simulink model "trial"  (R2020b)
settings: Solver=VariableStepAuto  StartTime=0.0  StopTime=10.0  RelTol=1e-3
libraries: simulink x2
settings Model: Creator=99003785  LastModifiedBy=99003785

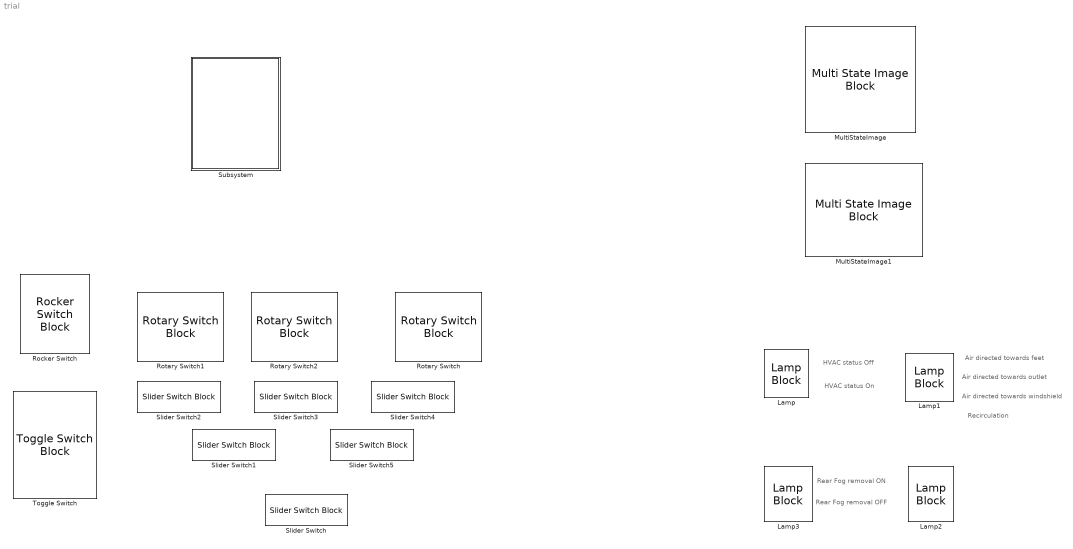
== system trial ==
  note: Rear Fog removal OFF
  note: Recirculation
  note: Air directed towards feet
  note: Air directed towards outlet
  note: Air directed towards windshield
  note: HVAC status On
  note: Rear Fog removal ON
  note: HVAC status Off
  Lamp{,1..3} (4 alike) : LampBlock
  MultiStateImage : MultiStateImageBlock
  MultiStateImage1 : MultiStateImageBlock
  Rocker Switch : RockerSwitchBlock
      settings: Values={{'On', 'Off'}, [1 0]}
  Rotary Switch : RotarySwitchBlock
      settings: Values={{'Off', 'Low', 'Medium', 'High'}, [0 1 2 3]}
  Rotary Switch1 : RotarySwitchBlock
      settings: Values={{'Off', 'Low', 'Medium', 'High'}, [0 1 2 3]}
  Rotary Switch2 : RotarySwitchBlock
      settings: Values={{'Off', 'AC', 'Heater', 'Air-Vent'}, [0 1 2 3]}
  Slider Switch{,1..5} (6 alike) : SliderSwitchBlock
      settings: Values={{'Off', 'On'}, [0 1]}
  Subsystem : Subsystem
  Toggle Switch : ToggleSwitchBlock
      settings: Values={{'Off', 'On'}, [0 1]}

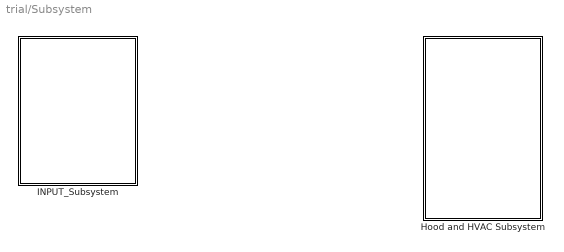
== system trial/Subsystem ==
  Hood and HVAC Subsystem : Subsystem  TreatAsAtomicUnit=on
  INPUT_Subsystem : Subsystem

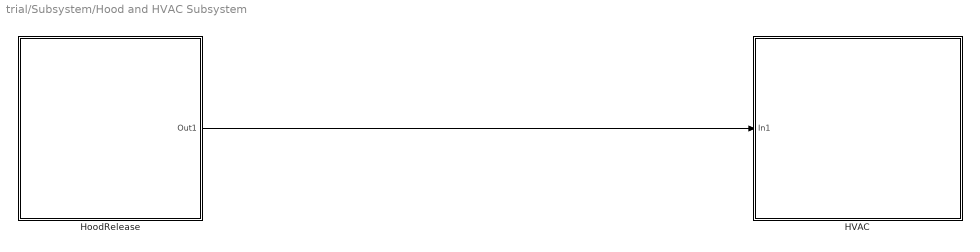
== system trial/Subsystem/Hood and HVAC Subsystem ==
  HVAC : Subsystem
  HoodRelease : Subsystem
  wires:
  HoodRelease/1(Out1) -> HVAC/1(In1)

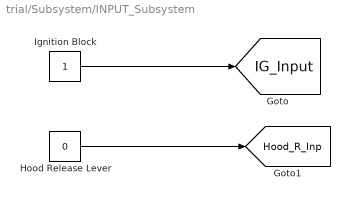
== system trial/Subsystem/INPUT_Subsystem ==
  Hood Release Lever : Constant  Value=0
  Ignition Block : Constant
  tag scope: Hood_R_Inp=global, IG_Input=global
  wires:
  Ignition Block/1 -> [IG_Input]
  Hood Release Lever/1 -> [Hood_R_Inp]

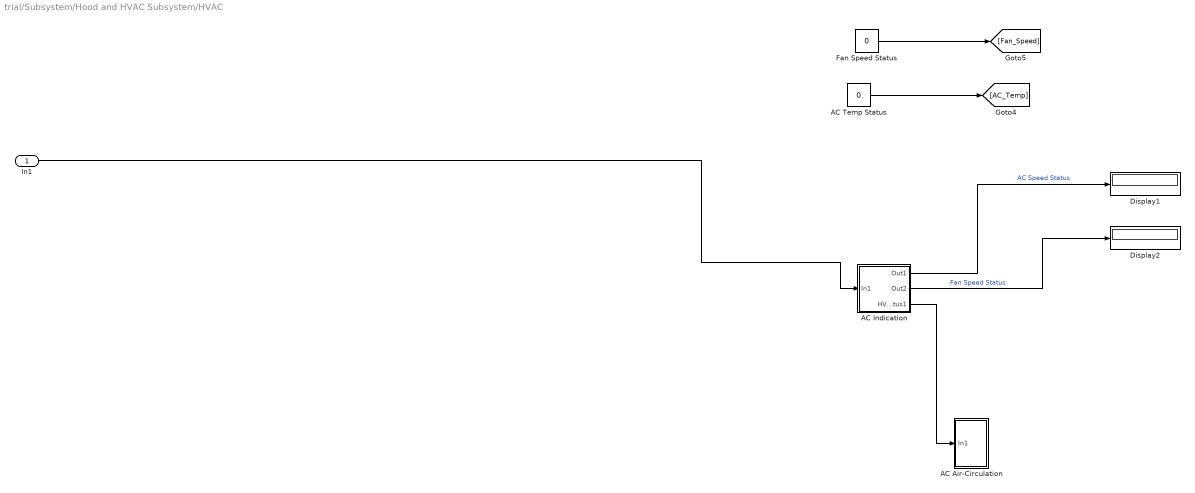
== system trial/Subsystem/Hood and HVAC Subsystem/HVAC ==
  In1 : Inport
  AC Air-Circulation : Subsystem
  AC Indication : Subsystem
  AC Temp Status : Constant  Value=0
  Display1 : Display
  Display2 : Display
  Fan Speed Status : Constant  Value=0
  wires:
  In1/1 -> AC Indication/1(In1)
  AC Indication/1(Out1) -> Display1/1  "AC Speed Status"
  AC Indication/2(Out2) -> Display2/1  "Fan Speed Status"
  AC Indication/3(HVAC Status1) -> AC Air-Circulation/1(In1)
  Fan Speed Status/1 -> [Fan_Speed]
  AC Temp Status/1 -> [AC_Temp]

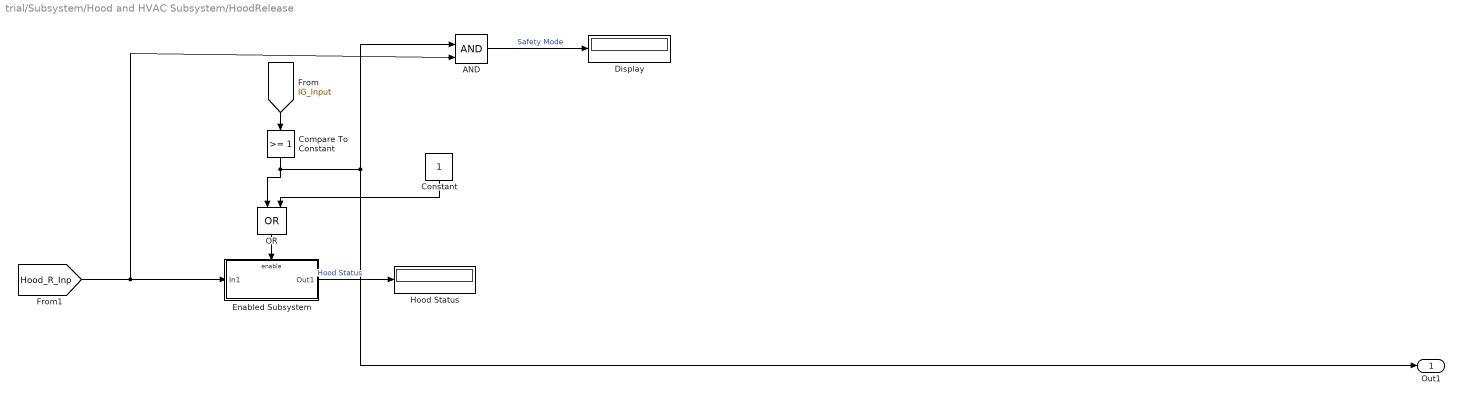
== system trial/Subsystem/Hood and HVAC Subsystem/HoodRelease ==
  AND : Logic  IconShape=distinctive  AllPortsSameDT=off  OutDataTypeStr=boolean
  Compare To Constant : simulink/Logic and Bit Operations/Compare To Constant  relop=>=  const=1  OutDataTypeStr=boolean
  Constant : Constant
  Display : Display
  Enabled Subsystem : Subsystem  TreatAsAtomicUnit=on
  Hood Status : Display
  OR : Logic  Operator=OR  IconShape=distinctive  AllPortsSameDT=off  OutDataTypeStr=boolean
  Out1 : Outport
  wires:
  [Hood_R_Inp] -> AND/2, Enabled Subsystem/1(In1)
  Enabled Subsystem/1(Out1) -> Hood Status/1  "Hood Status"
  Constant/1 -> OR/2
  OR/1 -> Enabled Subsystem/Enable
  AND/1 -> Display/1  "Safety Mode"
  [IG_Input] -> Compare To Constant/1
  Compare To Constant/1 -> Out1/1, AND/1, OR/1

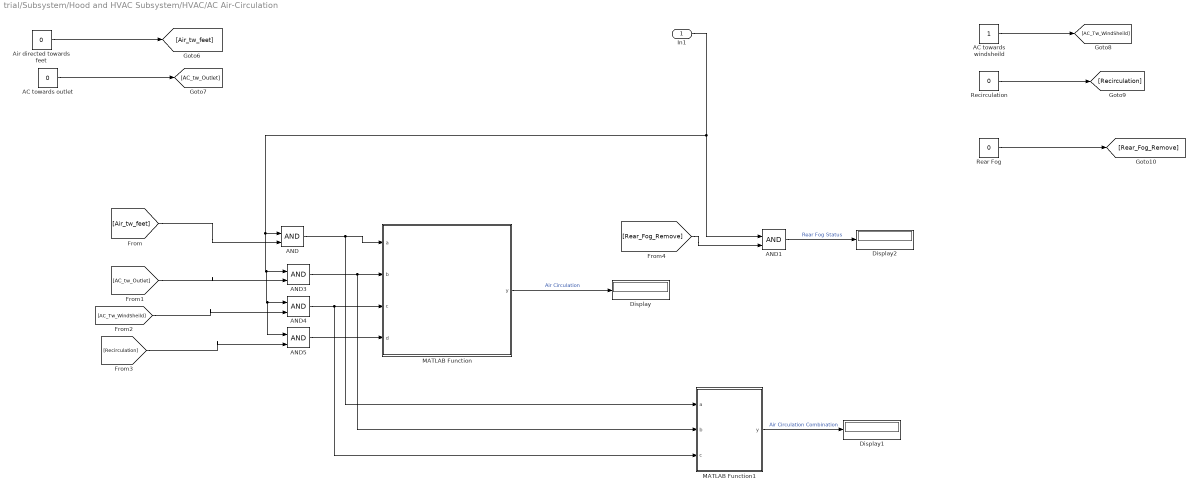
== system trial/Subsystem/Hood and HVAC Subsystem/HVAC/AC Air-Circulation ==
  In1 : Inport
  AC towards outlet : Constant  Value=0
  AC towards windsheild : Constant
  AND{,1,3..5} (5 alike) : Logic  IconShape=distinctive  AllPortsSameDT=off  OutDataTypeStr=boolean
  Air directed towards feet : Constant  Value=0
  Display : Display
  Display1 : Display
  Display2 : Display
  MATLAB Function : MATLAB Function  TreatAsAtomicUnit=on
  MATLAB Function1 : MATLAB Function  TreatAsAtomicUnit=on
  Rear Fog : Constant  Value=0
  Recirculation : Constant  Value=0
  wires:
  [AC_tw_Outlet] -> AND3/2
  In1/1 -> AND1/1, AND5/1, AND4/1, AND3/1, AND/1
  AND4/1 -> MATLAB Function1/3(c), MATLAB Function/3(c)
  MATLAB Function/1(y) -> Display/1  "Air Circulation"
  AND/1 -> MATLAB Function1/1(a), MATLAB Function/1(a)
  AND3/1 -> MATLAB Function1/2(b), MATLAB Function/2(b)
  AND5/1 -> MATLAB Function/4(d)
  [Air_tw_feet] -> AND/2
  MATLAB Function1/1(y) -> Display1/1  "Air Circulation Combination"
  [Rear_Fog_Remove] -> AND1/2
  AND1/1 -> Display2/1  "Rear Fog Status"
  [AC_Tw_WindSheild] -> AND4/2
  [Recirculation] -> AND5/2
  Air directed towards feet/1 -> [Air_tw_feet]
  AC towards outlet/1 -> [AC_tw_Outlet]
  Rear Fog/1 -> [Rear_Fog_Remove]
  Recirculation/1 -> [Recirculation]
  AC towards windsheild/1 -> [AC_Tw_WindSheild]

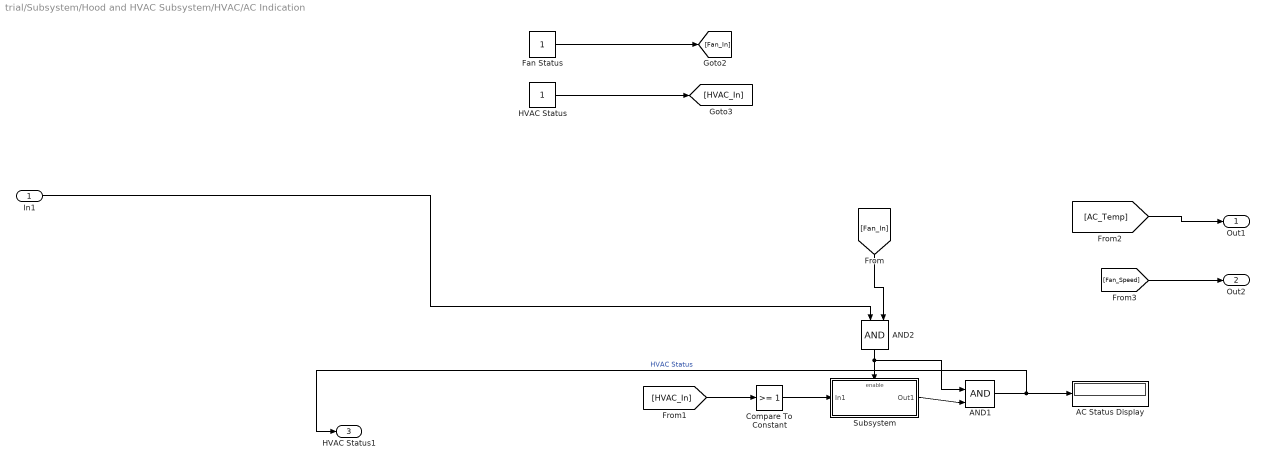
== system trial/Subsystem/Hood and HVAC Subsystem/HVAC/AC Indication ==
  In1 : Inport
  AC Status Display : Display
  AND1 : Logic  IconShape=distinctive  AllPortsSameDT=off  OutDataTypeStr=boolean
  AND2 : Logic  IconShape=distinctive  AllPortsSameDT=off  OutDataTypeStr=boolean
  Compare To Constant : simulink/Logic and Bit Operations/Compare To Constant  relop=>=  const=1  OutDataTypeStr=boolean
  Fan Status : Constant
  HVAC Status : Constant
  Subsystem : Subsystem
  Out1 : Outport
  Out2 : Outport  Port=2
  HVAC Status1 : Outport  Port=3
  wires:
  In1/1 -> AND2/1
  [Fan_Speed] -> Out2/1
  AND2/1 -> AND1/1, Subsystem/Enable
  Subsystem/1(Out1) -> AND1/2
  AND1/1 -> HVAC Status1/1, AC Status Display/1  "HVAC Status"
  [AC_Temp] -> Out1/1
  [HVAC_In] -> Compare To Constant/1
  Compare To Constant/1 -> Subsystem/1(In1)
  [Fan_In] -> AND2/2
  Fan Status/1 -> [Fan_In]
  HVAC Status/1 -> [HVAC_In]

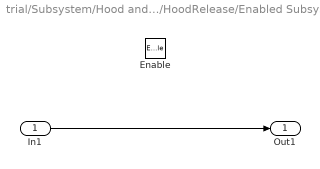
== system trial/Subsystem/Hood and HVAC Subsystem/HoodRelease/Enabled Subsystem ==
  In1 : Inport
  Enable : EnablePort
  Out1 : Outport  InitialOutput=0  VectorParamsAs1DForOutWhenUnconnected=off
  wires:
  In1/1 -> Out1/1

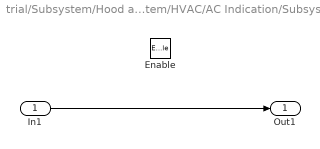
== system trial/Subsystem/Hood and HVAC Subsystem/HVAC/AC Indication/Subsystem ==
  In1 : Inport
  Enable : EnablePort
  Out1 : Outport
  wires:
  In1/1 -> Out1/1

== matlab function trial/Subsystem/Hood and HVAC Subsystem/HVAC/AC Air-Circulation/MATLAB Function1 ==
  data: a input; b input; c input; y output
function y = fcn(a,b,c)
    if a==1&& b==1 && c==1
        y=1;
    elseif a==1 && b==1 && c==0
        y=2;
    elseif a==1 && b==0 && c==1
        y=3;
    elseif a==0 && b==1 && c==1
        y=4;
    else
        y=0;
    end

end

== matlab function trial/Subsystem/Hood and HVAC Subsystem/HVAC/AC Air-Circulation/MATLAB Function ==
  data: a input; b input; y output; c input; d input
function y = fcn(a, b, c, d)
    if a==1 && b==0 && c==0 && d==0
        y=1;
    elseif a==0 && b==1 &&c==0 && d==0
        y=2;
    elseif a==0 && b==0 &&c==1 && d==0
        y=3;
    elseif a==0 && b==0 &&c==0 && d==1
        y=4;
    else
        y=0;
    end
    

end
